simulink model "blackhawk_3dof"  (Simulink 7.0)
settings: Solver=ode23  StartTime=0.0  StopTime=2  RelTol=1e-3
values from neighbouring files (symbols this model uses):
  a = 10*wd    [HelicopterHoverExample.m]
  Kden = [A1 A0]    [HelicopterHoverExample.m]
  Knum = [B1 B0]    [HelicopterHoverExample.m]
undefined symbols (not defined in the file or in its folder): plant_den, plant_num
settings Model: Creator=gabe  LastModifiedBy=gabe

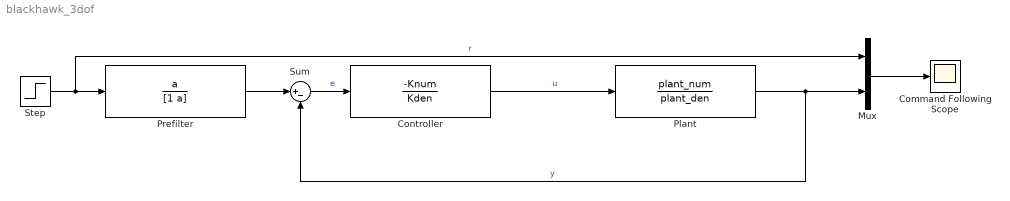
== system blackhawk_3dof ==
  Command Following Scope : Scope
      settings: TimeRange=2  YMin=0  YMax=1.5  SaveName=Pitch  SampleInput=on  SampleTime=1/10000
  Controller : TransferFcn  Numerator=-Knum  Denominator=Kden
  Mux : Mux  Inputs=2
  Plant : TransferFcn  Numerator=plant_num  Denominator=plant_den
  Prefilter : TransferFcn  Numerator=a  Denominator=[1 a]
  Step : Step  Time=0.25  SampleTime=0
  Sum : Sum  Inputs=|+-  OutDataType=sfix(16)  OutScaling=2^0
  wires:
  Plant/1 -> Mux/2, Sum/2  "y"
  Controller/1 -> Plant/1  "u"
  Step/1 -> Mux/1, Prefilter/1  "r"
  Sum/1 -> Controller/1  "e"
  Mux/1 -> Command Following Scope/1
  Prefilter/1 -> Sum/1
